simulink model "send_signal"  (R2017b)
settings: Solver=ode3  StartTime=0.0  StopTime=inf  FixedStep=0.01  RelTol=1e-3  EnableMultiTasking=on
InitFcn:
  | cutFreq = 0.1; % T
  | sampleTime = 0.01;
  | filt = tf(1,[cutFreq 1]);
  | filt = c2d(filt,sampleTime);
  | 
  | cutFreq2 = 1;
  | filt2 = tf(1,[cutFreq2 1]);
  | filt2 = c2d(filt2,sampleTime);
  | 
  | update_param = 1;
  | 
  | ampliFactor = 1.60;
  | ampliFactorMiddle = 2.00;
  | ampliFactorDistal = 1;
  | 
  | % Set Hand Address
  | RightHandAddress = '10.100.39.144';
  | Verosim = '10.100.39.22'
  | LeftHandAddress = '10.100.39.22'
model workspace (MAT data in the model file):
  SL_ROS_VariableLengthArrays_MaxSizes.CommonInfo.ArrayTruncateAction = 'EmitWarning'
  SL_ROS_VariableLengthArrays_MaxSizes.MsgTypeMap = containers.Map
  SL_ROS_VariableLengthArrays_MaxSizes.MsgTypeMap.serialization.keys = {'std_msgs/Float32MultiArray'}
  SL_ROS_VariableLengthArrays_MaxSizes.MsgTypeMap.serialization.values{1}.PropertyName = 'Data'
  SL_ROS_VariableLengthArrays_MaxSizes.MsgTypeMap.serialization.values{1}.DataType = 'single'
  SL_ROS_VariableLengthArrays_MaxSizes.MsgTypeMap.serialization.values{1}.MaxLength = 2
  SL_ROS_VariableLengthArrays_MaxSizes.MsgTypeMap.serialization.uniformity = 0
  SL_ROS_VariableLengthArrays_MaxSizes.MsgTypeMap.serialization.keyType = 'char'
  SL_ROS_VariableLengthArrays_MaxSizes.MsgTypeMap.serialization.valueType = 'any'
libraries: etargetslib x2, dspnetwork x2
settings Model: Creator=Centauro  LastModifiedBy=Tonno
settings DataIOCC: LimitDataPoints=on  SaveFormat=Array
settings OptimizationCC: PassReuseOutputArgsThreshold=0  MaxStackSize=64
settings DebuggingCC: ParameterTunabilityLossMsg=error  SFUnexpectedBacktrackingDiag=warning  SFNoUnconditionalDefaultTransitionDiag=warning  SFExecutionAtInitializationDiag=none
settings HardwareCC: ProdBitPerPointer=32  ProdBitPerSizeT=32  ProdBitPerPtrDiffT=32  ProdLargestAtomicFloat=None  ProdIntDivRoundTo=Undefined  ProdEndianess=Unspecified  ProdWordSize=32  ProdHWDeviceType=Generic->Unspecified (assume 32-bit Generic)  UseEmbeddedCoderFeatures=off
settings ModelReferenceCC: PropagateSignalLabelsOutOfModel=off
settings SFSimCC: MATLABDynamicMemAlloc=off
settings RTWCC: SystemTargetFile=ert.tlc  HardwareBoard=Robot Operating System (ROS)  TemplateMakefile=ert_default_tmf  GenerateReport=on  Toolchain=Catkin  LaunchReport=on  TargetLang=C++
settings CodeAppCC: ForceParamTrailComments=on  OperatorAnnotations=on
settings ERTTargetCC: ERTCustomFileBanners=off  SupportContinuousTime=on  SupportNonInlinedSFcns=on  RemoveResetFunc=off  ModelStepFunctionPrototypeControlCompliant=off
settings ConfigComp: CovMetricSettings=dw  CovHtmlReporting=on  CovSaveCumulativeToWorkspaceVar=on  CovSaveSingleToWorkspaceVar=on  CovExternalEMLEnable=off

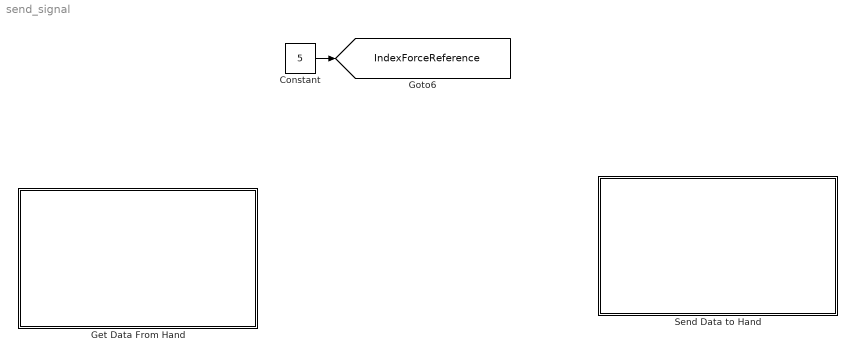
== system send_signal ==
  Constant : Constant  Value=5  OutDataTypeStr=single
  Get Data From Hand : Subsystem
  Send Data to Hand : Subsystem
  tag scope: IndexForceReference=global
  wires:
  Constant/1 -> [IndexForceReference]

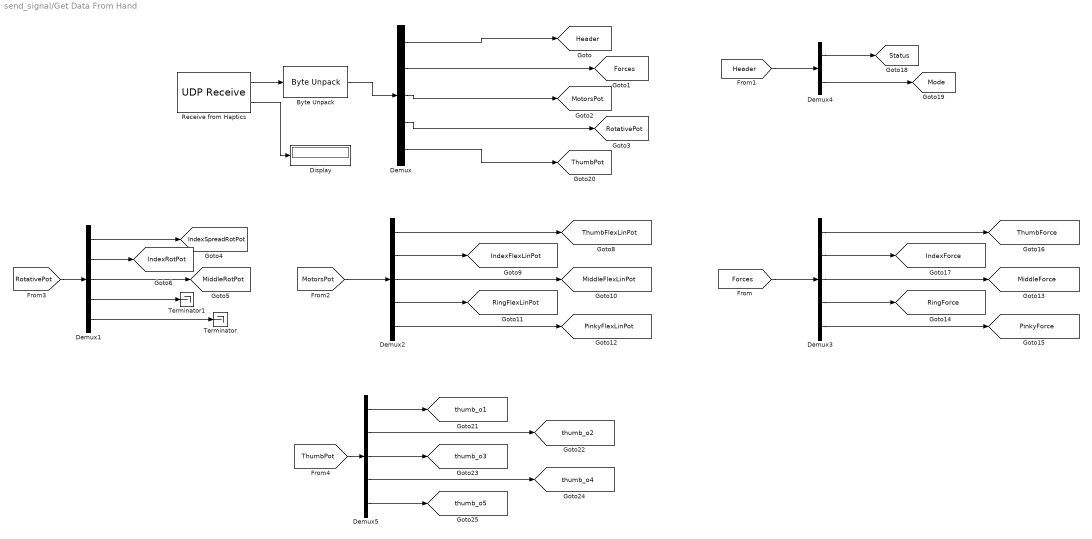
== system send_signal/Get Data From Hand ==
  Byte Unpack : etargetslib/Byte Unpack  dimensions={[22]}  datatypes={'single'}  byteAlign=1
  Demux : Demux  Outputs=[2, 5, 5, 5,5]
  Demux{1..3,5} (4 alike) : Demux  Outputs=5
  Demux4 : Demux  Outputs=2
  Display : Display
  Receive from Haptics : dspnetwork/UDP Receive  localURL='0.0.0.0'  localPort=15001  remoteURL='0.0.0.0'  remotePort=-1  recvBufferSize=22*4  dims=22*4  signalDatatype=uint8  isVarSize=off  showBlockingTime=on  blockingTime=inf  sampletime=0.01  blockPlatform=HOST
      settings: SourceProductName=DSP System Toolbox  SourceProductBaseCode=DS
  Terminator : Terminator
  Terminator1 : Terminator
  tag scope: Forces=global, Header=global, IndexFlexLinPot=global, IndexForce=global, IndexRotPot=global, IndexSpreadRotPot=global, MiddleFlexLinPot=global, MiddleForce=global, MiddleRotPot=global, Mode=global, MotorsPot=global, PinkyFlexLinPot=global, PinkyForce=global, RingFlexLinPot=global, RingForce=global, RotativePot=global, Status=global, ThumbFlexLinPot=global, ThumbForce=global, ThumbPot=global, thumb_o1=global, thumb_o2=global, thumb_o3=global, thumb_o4=global, thumb_o5=global
  wires:
  Demux/3 -> [MotorsPot]
  Demux/1 -> [Header]
  Demux/4 -> [RotativePot]
  Demux/2 -> [Forces]
  Receive from Haptics/2 -> Display/1
  [RotativePot] -> Demux1/1
  Demux1/2 -> [IndexRotPot]
  Demux1/3 -> [MiddleRotPot]
  Demux1/4 -> Terminator1/1
  Demux1/5 -> Terminator/1
  Demux1/1 -> [IndexSpreadRotPot]
  Demux2/1 -> [ThumbFlexLinPot]
  Demux2/2 -> [IndexFlexLinPot]
  [MotorsPot] -> Demux2/1
  Demux2/3 -> [MiddleFlexLinPot]
  Demux2/4 -> [RingFlexLinPot]
  Demux2/5 -> [PinkyFlexLinPot]
  Demux3/1 -> [ThumbForce]
  Demux3/2 -> [IndexForce]
  [Forces] -> Demux3/1
  Demux3/3 -> [MiddleForce]
  Demux3/4 -> [RingForce]
  Demux3/5 -> [PinkyForce]
  [Header] -> Demux4/1
  Demux4/1 -> [Status]
  Demux4/2 -> [Mode]
  Byte Unpack/1 -> Demux/1
  Receive from Haptics/1 -> Byte Unpack/1
  Demux/5 -> [ThumbPot]
  [ThumbPot] -> Demux5/1
  Demux5/1 -> [thumb_o1]
  Demux5/2 -> [thumb_o2]
  Demux5/3 -> [thumb_o3]
  Demux5/4 -> [thumb_o4]
  Demux5/5 -> [thumb_o5]

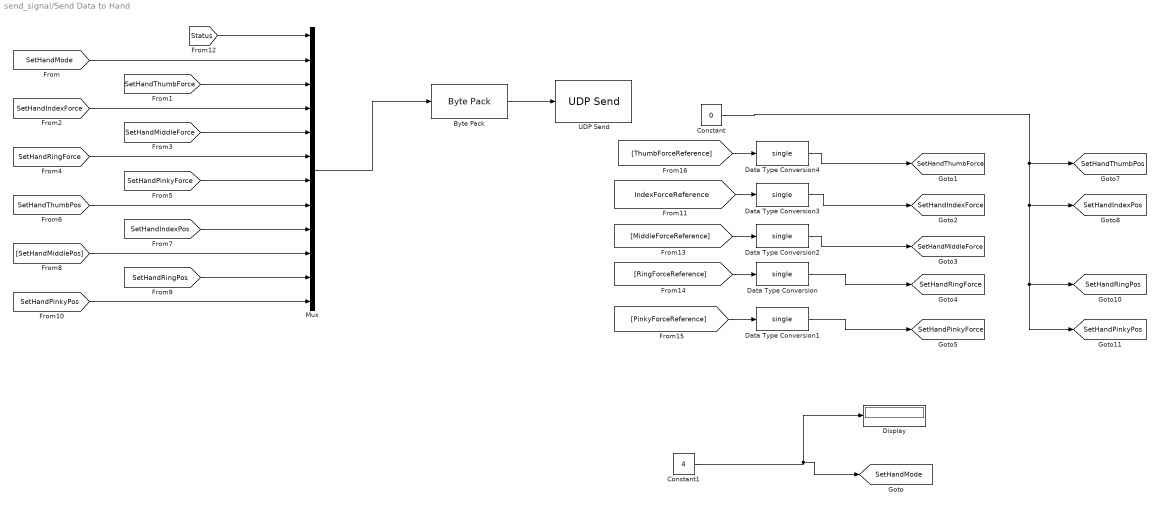
== system send_signal/Send Data to Hand ==
  Byte Pack : etargetslib/Byte Pack  datatypes={'single'}  byteAlign=1
  Constant : Constant  Value=0  OutDataTypeStr=single
  Constant1 : Constant  Value=4  OutDataTypeStr=single
  Data Type Conversion{,1..4} (5 alike) : DataTypeConversion  OutDataTypeStr=single
  Display : Display
  Mux : Mux  Inputs=12
  UDP Send : dspnetwork/UDP Send  remoteURL=RightHandAddress  remotePort=12000  localURL='0.0.0.0'  localPortSource=Automatically determine  localPort=-1  sampletime=-1  blockPlatform=HOST  separateLengthPort=0
      settings: SourceProductName=DSP System Toolbox  SourceProductBaseCode=DS
  tag scope: SetHandIndexForce=global, SetHandIndexPos=global, SetHandMiddleForce=global, SetHandMode=global, SetHandPinkyForce=global, SetHandPinkyPos=global, SetHandRingForce=global, SetHandRingPos=global, SetHandThumbForce=global, SetHandThumbPos=global
  wires:
  Byte Pack/1 -> UDP Send/1
  [SetHandMode] -> Mux/2
  [SetHandThumbForce] -> Mux/3
  [SetHandIndexForce] -> Mux/4
  [SetHandRingForce] -> Mux/6
  [SetHandMiddleForce] -> Mux/5
  [SetHandPinkyForce] -> Mux/7
  [SetHandThumbPos] -> Mux/8
  [SetHandIndexPos] -> Mux/9
  [SetHandMiddlePos] -> Mux/10
  [SetHandRingPos] -> Mux/11
  [SetHandPinkyPos] -> Mux/12
  [Status] -> Mux/1
  [ThumbForceReference] -> Data Type Conversion4/1
  [RingForceReference] -> Data Type Conversion/1
  [PinkyForceReference] -> Data Type Conversion1/1
  [MiddleForceReference] -> Data Type Conversion2/1
  [IndexForceReference] -> Data Type Conversion3/1
  Constant/1 -> [SetHandThumbPos], [SetHandIndexPos], [SetHandRingPos], [SetHandPinkyPos]
  Mux/1 -> Byte Pack/1
  Data Type Conversion/1 -> [SetHandRingForce]
  Data Type Conversion1/1 -> [SetHandPinkyForce]
  Data Type Conversion2/1 -> [SetHandMiddleForce]
  Data Type Conversion3/1 -> [SetHandIndexForce]
  Data Type Conversion4/1 -> [SetHandThumbForce]
  Constant1/1 -> [SetHandMode], Display/1
